simulink model "StateFeedbackK"  (R2023a)
settings: Solver=VariableStepAuto  StartTime=0.0  StopTime=10  RelTol=1e-3
undefined symbols (not defined in the file): A_1, B_1_Ajuste, C_1, K, Lc_corrige
settings Model: Creator=orvik  LastModifiedBy=orvik

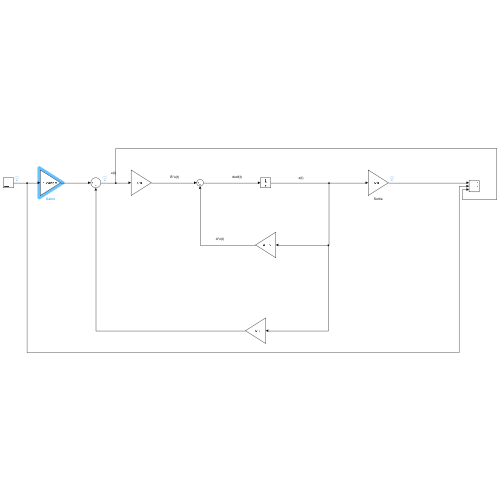
[thumbnail: Simulink's stored preview of the top-level diagram]
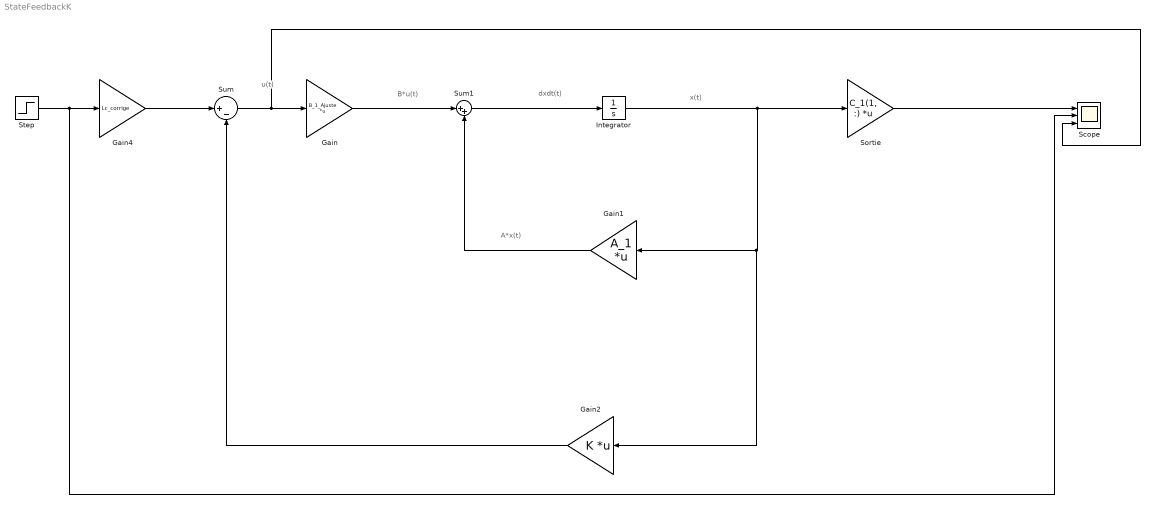
== system StateFeedbackK ==
  note: u(t)
  note: B*u(t)
  note: A*x(t)
  note: x(t)
  note: dxdt(t)
  Gain : Gain  Gain=B_1_Ajuste  Multiplication=Matrix(K*u)
  Gain1 : Gain  Gain=A_1  Multiplication=Matrix(K*u)
  Gain2 : Gain  Gain=K  Multiplication=Matrix(K*u)
  Gain4 : Gain  Gain=Lc_corrige
  Integrator : Integrator
  Scope : Scope  NumInputPorts=3
  Sortie : Gain  Gain=C_1(1, :)  Multiplication=Matrix(K*u)
  Step : Step  After=pi/5  SampleTime=0
  Sum : Sum  Inputs=|+-
  Sum1 : Sum  Inputs=|++
  wires:
  Gain/1 -> Sum1/1
  Integrator/1 -> Gain2/1, Gain1/1, Sortie/1
  Gain1/1 -> Sum1/2
  Step/1 -> Scope/2, Gain4/1
  Sum/1 -> Scope/3, Gain/1
  Gain4/1 -> Sum/1
  Sum1/1 -> Integrator/1
  Sortie/1 -> Scope/1
  Gain2/1 -> Sum/2
